simulink model "cruise_model_open_loop"  (R2024a)
settings: Solver=VariableStepAuto  StartTime=0.0  StopTime=700  RelTol=1e-3
settings Model: Creator=root  LastModifiedBy=kiran m v
settings SolverCC: AlgebraicLoopSolver=TrustRegion
settings DataIOCC: ReturnWorkspaceOutputs=off
settings DebuggingCC: UnconnectedInputMsg=warning  UnconnectedOutputMsg=warning  UnconnectedLineMsg=warning  ArithmeticOperatorsInVariantConditions=warning
settings ModelReferenceCC: EnableRefExpFcnMdlSchedulingChecks=on
settings SFSimCC: SimUseLocalCustomCode=off  CustomCodeUndefinedFunction=UseInterfaceOnly
settings RTWCC: RTWUseLocalCustomCode=off  GPUComputeCapability=3.5
settings CodeAppCC: StateflowObjectComments=on

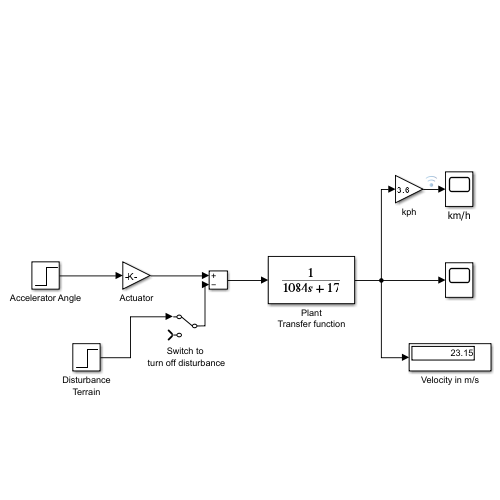
[thumbnail: Simulink's stored preview of the top-level diagram]
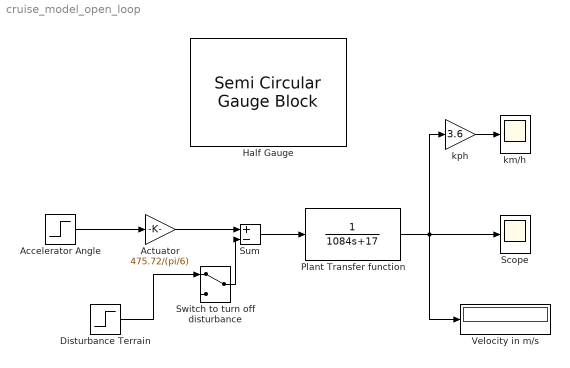
== system cruise_model_open_loop ==
  Accelerator Angle : Step  After=pi/6  SampleTime=0
  Actuator : Gain  Gain=475.72/(pi/6)
  Disturbance Terrain : Step  Time=350  After=475.72*9.81*sin(pi/45)  SampleTime=0
  Half Gauge : SemiCircularGaugeBlock  ScaleMax=220
  Plant Transfer function : TransferFcn  Denominator=[1084 17]
  Scope : Scope
  Sum : Sum  Inputs=+-
  Switch to turn off disturbance : ManualSwitch
  Velocity in m/s : Display
  km/h : Scope
  kph : Gain  Gain=3.6
  wires:
  Accelerator Angle/1 -> Actuator/1
  Plant Transfer function/1 -> Velocity in m/s/1, kph/1, Scope/1
  kph/1 -> km/h/1
  Actuator/1 -> Sum/1
  Sum/1 -> Plant Transfer function/1
  Disturbance Terrain/1 -> Switch to turn off disturbance/1
  Switch to turn off disturbance/1 -> Sum/2
